simulink model "plant_model"  (R2021a)
settings: Solver=VariableStepAuto  StartTime=0.0  StopTime=10.0  RelTol=1e-3
undefined symbols (not defined in the file): BMSBatteryPackData, BMSContactorModuleData, BusSOCEstimation, ChargerCurrent, ChargerVoltage, IBatt, ICharger, IInverter, InverterCurrent, InverterVoltage, SegmentCurrentVector, SegmentRealSOCVector, SegmentTempVector, SegmentVoltageVector, SimulationChargerData, SimulationInverterData, VBatt, VCharger, VInverter
libraries: fl_lib x1, nesl_utility x1
settings Model: Creator=Carlo Edoardo  LastModifiedBy=miche

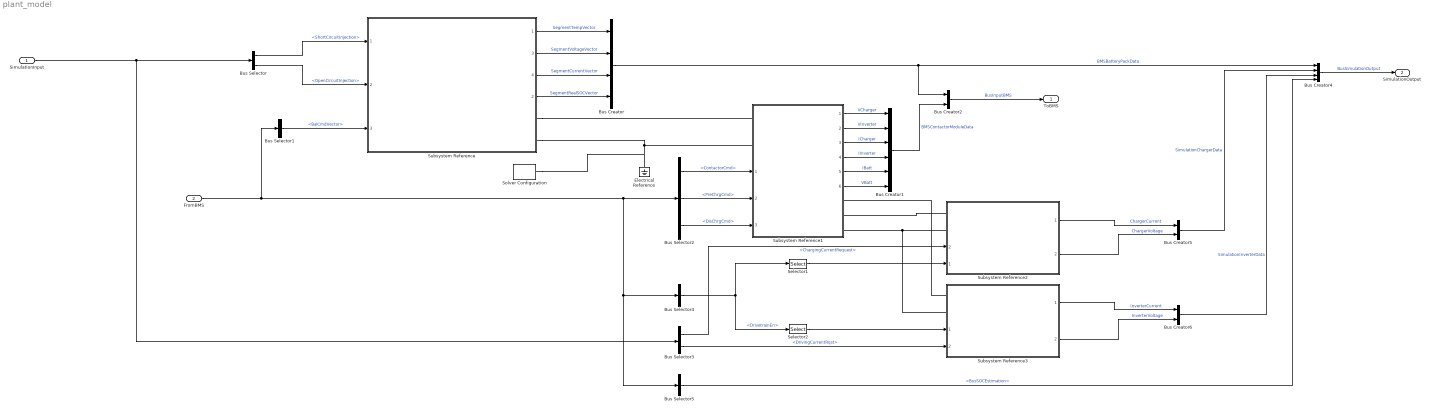
== system plant_model ==
  SimulationInput : Inport  OutDataTypeStr=Bus: BusSimulationInput
  FromBMS : Inport  Port=2  OutDataTypeStr=Bus: BusOutputBMS
  Bus Creator : BusCreator  Inputs=SegmentTempVector,SegmentVoltageVector,SegmentCurrentVector,SegmentRealSOCVector  OutDataTypeStr=Bus: BMSBatteryPackData
  Bus Creator1 : BusCreator  Inputs=VCharger,VInverter,ICharger,IInverter,IBatt,VBatt  OutDataTypeStr=Bus: BMSContactorModuleData
  Bus Creator2 : BusCreator  Inputs=BMSBatteryPackData,BMSContactorModuleData  OutDataTypeStr=Bus: BusInputBMS
  Bus Creator4 : BusCreator  Inputs=BMSBatteryPackData,SimulationChargerData,SimulationInverterData,BusSOCEstimation  OutDataTypeStr=Bus: BusSimulationOutput
  Bus Creator5 : BusCreator  Inputs=ChargerCurrent,ChargerVoltage  OutDataTypeStr=Bus: SimulationChargerData
  Bus Creator6 : BusCreator  Inputs=InverterCurrent,InverterVoltage  OutDataTypeStr=Bus: SimulationInverterData
  Bus Selector : BusSelector  OutputSignals=SimulationBatteryPackInput.ShortCircuitInjection,SimulationBatteryPackInput.OpenCircuitInjection
  Bus Selector1 : BusSelector  OutputSignals=BMSBatteryPackInput.BalCmdVector
  Bus Selector2 : BusSelector  OutputSignals=BMSContactorModuleCmd.ContactorCmd,BMSContactorModuleCmd.PreChrgCmd,BMSContactorModuleCmd.DisChrgCmd
  Bus Selector3 : BusSelector  OutputSignals=SimulationSystemInput.ChargingCurrentRequest,SimulationSystemInput.DrivingCurrentRqst
  Bus Selector4 : BusSelector  OutputSignals=BMSContactorModuleCmd.DrivetrainEn
  Bus Selector5 : BusSelector  OutputSignals=BusSOCEstimation
  Electrical Reference : fl_lib/Electrical/Electrical Elements/Electrical Reference
  Selector1 : Selector  InputPortWidth=2  IndexOptions=Index vector (dialog)  Indices=1  OutputSizes=1
  Selector2 : Selector  InputPortWidth=2  IndexOptions=Index vector (dialog)  Indices=2  OutputSizes=1
  Solver Configuration : nesl_utility/Solver Configuration  PhysicalDomain=network_engine_domain  SubClassName=solver  LeftPortType=input  RightPortType=generic  Tones=[]  Harmonics=[]  SimulateNoise=off  Profile=off  UseLocalSampling=off  EnableSwitchedLinearOptims=on  FrequencyDomain=off  UseCCode=off  RelTol=0.001  AbsTol=1e-06  MinStep=1e-09  ToWorkspace=off  RevertToSquareIcSolve=off  NumHomotopyIterations=100  PhasorMode=off  PhasorModeNumHarmonics=1  DoDC=off  ResidualTolerance=1e-09  UseLocalSolver=off  LocalSolverChoice=NE_BACKWARD_EULER_ADVANCER  LocalSolverSampleTime=0.001  DoFixedCost=off  MaxNonlinIter=3  MaxModeIter=2  ComputeImpulses=off  ImpulseIterations=2  LinearAlgebra=auto  EquationFormulation=NE_TIME_EF  DelaysMemoryBudget=1024  AutomaticFiltering=on  FilteringTimeConstant=0.001  PartitionStorageMethod=AS_NEEDED  PartitionMemoryBudget=1024  PartitionMethod=ROBUST
      settings: SourceProductBaseCode=PW,SS
  Subsystem Reference : Subsystem  ReferencedSubsystem=battery_pack
      settings: PortSchema="{\"entries\":[{\"content\":{\"sides\":[{\"content\":{\"connectorIds\":[\"In1\",\"In2\",\"In3\"]},\"type\":\"ConnectorPlacement.EquallySpacedRectSide\",\"uuid\":\"a667b6fc-681b-4a6d-8bc5-1690d48ceb62\"},{\"content\":{\"connectorIds\":[\"Out1\",\"Out3\",\"Out4\",\"Out2\",\"RConn1\",\"RConn2\"],\"side\":\"RIGHT\"},\"type\":\"ConnectorPlacement.EquallySpacedRectSide\",\"uuid\":\"92bca01f-af96-4b42-a4ef-f99f9cfbda4a\"},{\"content\":{\"connectorIds\":[],\"side\":\"TOP\"},\"type\":\"ConnectorPlacement.EquallySpacedRectSide\",\"uuid\":\"1cddbf46-8c73-4905-947f-97e35e766652\"}]},\"type\":\"ConnectorPlacement.EquallySpacedConnector\",\"uuid\":\"4a3a4780-465f-41eb-aa1a-ebd0271dc245\"}],\"packageUris\":[\"http://schema.mathworks.com/mf0/Connector/R2020b\"],\"version\":\"1.0\"}"
  Subsystem Reference1 : Subsystem  ReferencedSubsystem=contactor_module
      settings: PortSchema="{\"entries\":[{\"content\":{\"sides\":[{\"content\":{\"connectorIds\":[\"LConn1\",\"LConn2\",\"In1\",\"In2\",\"In3\"]},\"type\":\"ConnectorPlacement.EquallySpacedRectSide\",\"uuid\":\"5963ee95-4cb8-4880-b10e-da21d6b626bd\"},{\"content\":{\"connectorIds\":[\"Out1\",\"Out2\",\"Out3\",\"Out4\",\"Out5\",\"Out6\",\"RConn2\",\"RConn1\",\"RConn3\"],\"side\":\"RIGHT\"},\"type\":\"ConnectorPlacement.EquallySpacedRectSide\",\"uuid\":\"9a40fd08-affa-4916-a7d8-056fd6ad8598\"},{\"content\":{\"connectorIds\":[],\"side\":\"TOP\"},\"type\":\"ConnectorPlacement.EquallySpacedRectSide\",\"uuid\":\"ee3c018e-d0a4-4c8f-9a3a-0084a0163dc4\"}]},\"type\":\"ConnectorPlacement.EquallySpacedConnector\",\"uuid\":\"fe72a94b-72d0-47f7-a7e4-1cbf8193dfc6\"}],\"packageUris\":[\"http://schema.mathworks.com/mf0/Connector/R2020b\"],\"version\":\"1.0\"}"
  Subsystem Reference2 : Subsystem  ReferencedSubsystem=battery_charger
      settings: PortSchema="{\"entries\":[{\"content\":{\"sides\":[{\"content\":{\"connectorIds\":[\"LConn1\",\"LConn2\",\"In2\",\"In1\"]},\"type\":\"ConnectorPlacement.EquallySpacedRectSide\",\"uuid\":\"fff7bc4f-531f-4bc4-8467-d658422a8955\"},{\"content\":{\"connectorIds\":[\"Out1\",\"Out2\"],\"side\":\"RIGHT\"},\"type\":\"ConnectorPlacement.EquallySpacedRectSide\",\"uuid\":\"a3b97e3b-e600-4156-97d8-d16c71fb8daf\"},{\"content\":{\"connectorIds\":[],\"side\":\"TOP\"},\"type\":\"ConnectorPlacement.EquallySpacedRectSide\",\"uuid\":\"2b5ac748-c7ee-4078-b49a-f9fdf4d626da\"}]},\"type\":\"ConnectorPlacement.EquallySpacedConnector\",\"uuid\":\"601ed575-6e2e-485e-997b-9ec3280c2b36\"}],\"packageUris\":[\"http://schema.mathworks.com/mf0/Connector/R2020b\"],\"version\":\"1.0\"}"
  Subsystem Reference3 : Subsystem  ReferencedSubsystem=drivetrain
      settings: PortSchema="{\"entries\":[{\"content\":{\"sides\":[{\"content\":{\"connectorIds\":[\"LConn1\",\"LConn2\",\"In1\",\"In2\"]},\"type\":\"ConnectorPlacement.EquallySpacedRectSide\",\"uuid\":\"67373542-6387-4049-a0c2-7d6efbd608a3\"},{\"content\":{\"connectorIds\":[\"Out1\",\"Out2\"],\"side\":\"RIGHT\"},\"type\":\"ConnectorPlacement.EquallySpacedRectSide\",\"uuid\":\"eadcaf5a-37e1-4626-99e2-0fa7c7540b07\"},{\"content\":{\"connectorIds\":[],\"side\":\"TOP\"},\"type\":\"ConnectorPlacement.EquallySpacedRectSide\",\"uuid\":\"47a838ef-809e-4a31-8207-6f2d1b789912\"}]},\"type\":\"ConnectorPlacement.EquallySpacedConnector\",\"uuid\":\"83c4aac4-981f-4b11-9d51-f7a7d8598d7f\"}],\"packageUris\":[\"http://schema.mathworks.com/mf0/Connector/R2020b\"],\"version\":\"1.0\"}"
  ToBMS : Outport  OutDataTypeStr=Bus: BusInputBMS
  SimulationOutput : Outport  Port=2  OutDataTypeStr=Bus: BusSimulationOutput
  wires:
  Subsystem Reference/1 -> Bus Creator/1  "SegmentTempVector"
  Subsystem Reference/3 -> Bus Creator/2  "SegmentVoltageVector"
  Subsystem Reference1/1 -> Bus Creator1/1  "VCharger"
  Subsystem Reference1/2 -> Bus Creator1/2  "VInverter"
  Subsystem Reference1/3 -> Bus Creator1/3  "ICharger"
  Subsystem Reference1/4 -> Bus Creator1/4  "IInverter"
  Subsystem Reference1/5 -> Bus Creator1/5  "IBatt"
  Subsystem Reference1/6 -> Bus Creator1/6  "VBatt"
  Bus Creator2/1 -> ToBMS/1  "BusInputBMS"
  SimulationInput/1 -> Bus Selector3/1, Bus Selector/1
  Bus Selector/1 -> Subsystem Reference/1  "<ShortCircuitInjection>"
  Bus Selector/2 -> Subsystem Reference/2  "<OpenCircuitInjection>"
  FromBMS/1 -> Bus Selector1/1, Bus Selector5/1, Bus Selector4/1, Bus Selector2/1
  Bus Selector1/1 -> Subsystem Reference/3  "<BalCmdVector>"
  Bus Selector2/1 -> Subsystem Reference1/1  "<ContactorCmd>"
  Bus Selector2/2 -> Subsystem Reference1/2  "<PreChrgCmd>"
  Bus Selector2/3 -> Subsystem Reference1/3  "<DisChrgCmd>"
  Bus Creator1/1 -> Bus Creator2/2  "BMSContactorModuleData"
  Bus Creator/1 -> Bus Creator2/1, Bus Creator4/1  "BMSBatteryPackData"
  Subsystem Reference/4 -> Bus Creator/3  "SegmentCurrentVector"
  Bus Creator4/1 -> SimulationOutput/1  "BusSimulationOutput"
  Bus Selector3/1 -> Subsystem Reference2/2  "<ChargingCurrentRequest>"
  Bus Selector3/2 -> Subsystem Reference3/2  "<DrivingCurrentRqst>"
  Subsystem Reference2/1 -> Bus Creator5/1  "ChargerCurrent"
  Subsystem Reference2/2 -> Bus Creator5/2  "ChargerVoltage"
  Subsystem Reference3/1 -> Bus Creator6/1  "InverterCurrent"
  Subsystem Reference3/2 -> Bus Creator6/2  "InverterVoltage"
  Bus Creator5/1 -> Bus Creator4/2  "SimulationChargerData"
  Bus Creator6/1 -> Bus Creator4/3  "SimulationInverterData"
  Selector1/1 -> Subsystem Reference2/1
  Selector2/1 -> Subsystem Reference3/1
  Bus Selector4/1 -> Selector1/1, Selector2/1  "<DrivetrainEn>"
  Subsystem Reference/2 -> Bus Creator/4  "SegmentRealSOCVector"
  Bus Selector5/1 -> Bus Creator4/4  "<BusSOCEstimation>"
  connections:
  Subsystem Reference/RConn1 -- Subsystem Reference1/LConn1
  Subsystem Reference/RConn2 -- Solver Configuration/RConn1 -- Electrical Reference/LConn1 -- Subsystem Reference1/LConn2
  Subsystem Reference2/LConn2 -- Subsystem Reference3/LConn2 -- Subsystem Reference1/RConn3
  Subsystem Reference2/LConn1 -- Subsystem Reference1/RConn1
  Subsystem Reference3/LConn1 -- Subsystem Reference1/RConn2
